simulink model "foucaultStart1"  (R2018b)
settings: Solver=ode23t  StartTime=0.0  StopTime=3600  FixedStep=.1  RelTol=1e-5  EnableMultiTasking=on
PreLoadFcn:
  | g = 9.83;          % acceleration of gravity (m/sec^2)
  | L = 67;            % pendulum length (m)
  | initial_x = L/100; % initial x coordinate (m)
  | initial_y = 0;     % initial y coordinate (m)
  | initial_xdot = 0;  % initial x velocity (m/sec)
  | initial_ydot = 0;  % initial y velocity (m/sec)
  | Omega=2*pi/86400;  % Earth's angular velocity of rotation about its axis (rad/sec)
  | lambda=49/180*pi;  % latitude in (rad)
CloseFcn:
  | close(findobj('Tag','CloseMe'));
settings Model: Creator=The MathWorks Inc.  LastModifiedBy=Alexander
settings DataIOCC: SaveFormat=StructureWithTime  SaveOutput=off  SaveTime=off  SignalLoggingName=sldemo_foucault_output
settings OptimizationCC: ExpressionDepthLimit=2147483647  InitFltsAndDblsToZero=on  LifeSpan=inf
settings DebuggingCC: SaveWithParameterizedLinksMsg=none  UnderspecifiedInitializationDetection=Classic  MergeDetectMultiDrivingBlocksExec=none  SignalResolutionControl=TryResolveAllWithWarning  ParameterPrecisionLossMsg=none  FcnCallInpInsideContextMsg=warning  AllowSymbolicDim=off  StateNameClashWarn=warning  LibraryContextMissingDiagnostic=none  SFUnexpectedBacktrackingDiag=warning  SFNoUnconditionalDefaultTransitionDiag=warning  SFExecutionAtInitializationDiag=none
settings HardwareCC: ProdBitPerPointer=32  ProdBitPerSizeT=32  ProdBitPerPtrDiffT=32  ProdLargestAtomicFloat=None  ProdIntDivRoundTo=Undefined  ProdEndianess=Unspecified  ProdWordSize=32  ProdHWDeviceType=32-bit Generic
settings ModelReferenceCC: PropagateSignalLabelsOutOfModel=off
settings SFSimCC: SimUseLocalCustomCode=off
settings RTWCC: RTWUseLocalCustomCode=off
settings CodeAppCC: StateflowObjectComments=on
settings GRTTargetCC: TargetFcnLib=ansi_tfl_tmw.mat  TargetLangStandard=C89/C90 (ANSI)  GeneratePreprocessorConditionals=Disable all  CombineOutputUpdateFcns=off  GRTInterface=on
settings ConfigComp: CovMetricSettings=dw  CovHtmlReporting=on  CovSaveCumulativeToWorkspaceVar=on  CovSaveSingleToWorkspaceVar=on  CovExternalEMLEnable=off  CovSFcnEnable=off

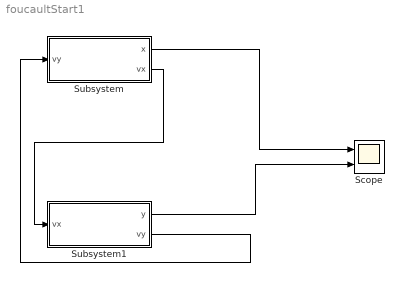
== system foucaultStart1 ==
  Scope : Scope  NumInputPorts=2
  Subsystem : Subsystem
  Subsystem1 : Subsystem
  wires:
  Subsystem/1(x) -> Scope/1
  Subsystem/2(vx) -> Subsystem1/1(vx)
  Subsystem1/2(vy) -> Subsystem/1("vy ")
  Subsystem1/1(y) -> Scope/2

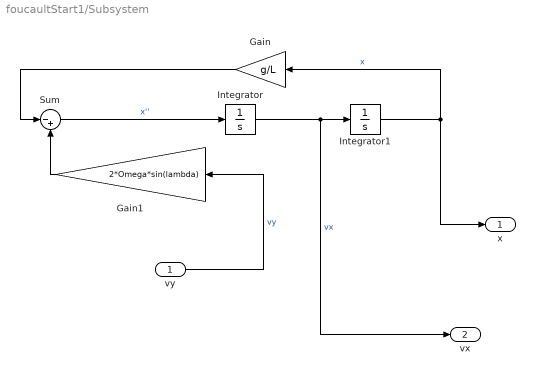
== system foucaultStart1/Subsystem ==
  "vy " : Inport
  Gain : Gain  Gain=g/L
  Gain1 : Gain  Gain=2*Omega*sin(lambda)
  Integrator : Integrator  InitialCondition=initial_xdot
  Integrator1 : Integrator  InitialCondition=initial_x
  Sum : Sum  Inputs=|-+
  x : Outport
  vx : Outport  Port=2
  wires:
  Gain1/1 -> Sum/2
  Integrator/1 -> vx/1, Integrator1/1  "vx"
  "vy "/1 -> Gain1/1  "vy"
  Gain/1 -> Sum/1
  Sum/1 -> Integrator/1  "x''"
  Integrator1/1 -> x/1, Gain/1  "x"

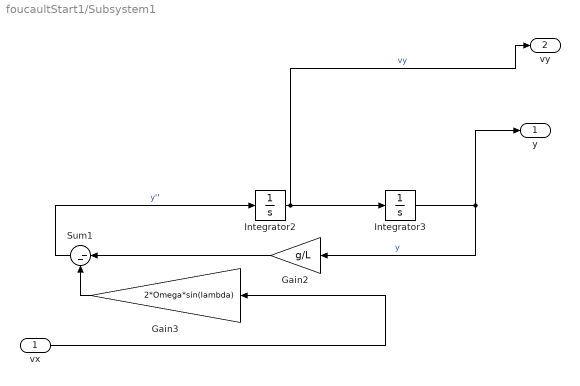
== system foucaultStart1/Subsystem1 ==
  vx : Inport
  Gain2 : Gain  Gain=g/L
  Gain3 : Gain  Gain=2*Omega*sin(lambda)
  Integrator2 : Integrator  InitialCondition=initial_ydot
  Integrator3 : Integrator  InitialCondition=initial_y
  Sum1 : Sum  Inputs=|--
  y : Outport
  vy : Outport  Port=2
  wires:
  vx/1 -> Gain3/1
  Sum1/1 -> Integrator2/1  "y''"
  Gain2/1 -> Sum1/1
  Integrator2/1 -> vy/1, Integrator3/1  "vy"
  Integrator3/1 -> y/1, Gain2/1  "y"
  Gain3/1 -> Sum1/2
